simulink model "gm_sampleModel2005_4_sub_sub"  (R2023a)
settings: Solver=VariableStepAuto  StartTime=0.0  StopTime=10.0  RelTol=1e-3
libraries: hdlsllib x5, simulink x1
settings Model: Creator=user1  LastModifiedBy=user1
settings OptimizationCC: BlockReduction=off  ConditionallyExecuteInputs=off
settings DebuggingCC: InheritedTsInSrcMsg=none

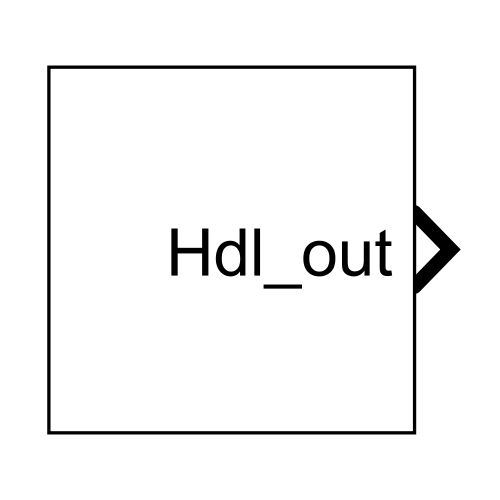
[thumbnail: Simulink's stored preview of the top-level diagram]
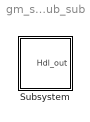
== system gm_sampleModel2005_4_sub_sub ==
  Subsystem : Subsystem

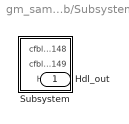
== system gm_sampleModel2005_4_sub_sub/Subsystem ==
  Subsystem : Subsystem
  Hdl_out : Outport  OutDataTypeStr=uint8

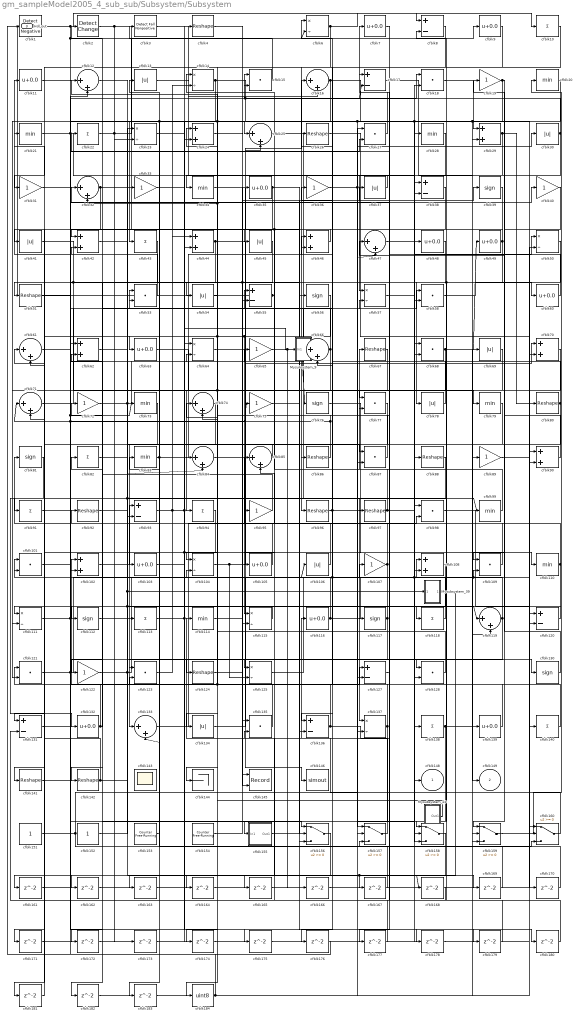
== system gm_sampleModel2005_4_sub_sub/Subsystem/Subsystem ==
  Mysubsystem_24 : Subsystem  TreatAsAtomicUnit=on  RTWFcnName=Mysubsystem_24
      settings: RTWFcnNameOpts=User specified  RTWFileNameOpts=Use function name
  Mysubsystem_39 : Subsystem  TreatAsAtomicUnit=on  RTWFcnName=Mysubsystem_39
      settings: RTWFcnNameOpts=User specified  RTWFileNameOpts=Use function name
  Mysubsystem_9 : Subsystem  TreatAsAtomicUnit=on  RTWFcnName=Mysubsystem_9
      settings: RTWFcnNameOpts=User specified  RTWFileNameOpts=Use function name
  cfblk1 : hdlsllib/Logic and Bit Operations/Detect Fall Negative  vinit=0  OutDataTypeStr=uint8
  cfblk{10,22,43,82,91,94,113,118,138,140} (10 alike) : Sum  Inputs=+  OutDataTypeStr=uint8
  cfblk{15,18,27,53,58,68,77,87,98,101,109,121,123,128,135} (15 alike) : DotProduct  OutDataTypeStr=uint8
  cfblk{24,29,42,44,46,62,70,90,102,108} (10 alike) : Sum  OutDataTypeStr=uint8
  cfblk{7,9,11,35,48..49,60,63,103,105,116,132,139} (13 alike) : Bias  Bias=0.0  SaturateOnIntegerOverflow=off
  cfblk{6,14,23,50,57,64,104,111,115,125,137} (11 alike) : Product  Inputs=*/  OutDataTypeStr=uint8  RndMeth=Zero  SaturateOnIntegerOverflow=on
  cfblk{13,30,37,41,45,54,69,78,106,134} (10 alike) : Abs  OutDataTypeStr=uint8  SaturateOnIntegerOverflow=off
  cfblk{19,31,33,36,40,65,72,75,89,95,107,122} (12 alike) : Gain  OutDataTypeStr=uint8
  cfblk{20..21,28,34,73,79,83,99,110,114} (10 alike) : MinMax  OutDataTypeStr=uint8
  cfblk{39,56,76,81,112,117,130} (7 alike) : Signum
  cfblk{12,16,25,32,47,61,66,71,74,84..85,119,133} (13 alike) : Sum  Inputs=|++  OutDataTypeStr=uint8
  cfblk{8,17,38,55,93,120,127,131,136} (9 alike) : Sum  Inputs=+-  OutDataTypeStr=uint8
  cfblk{4,26,51,67,80,86,88,92,96..97,124,141..142} (13 alike) : Reshape
  cfblk143 : Scope
      settings: Floating=on
  cfblk144 : Terminator
  cfblk145 : Record  FileSettingsInternal="{\"entries\":[{\"content\":{\"excelSettings\":{\"content\":{},\"type\":\"Streamout.ExcelSettings\"}},\"type\":\"Streamout.FileSettingStorage\",\"uuid\":\"\"}],\"packageUris\":[\"http:\\/\\/schema.mathworks.com\\/mf0\\/streamout_blocks\\/R2020a\"],\"version\":\"1.0\"}"  Layout=[1 1]  SignalsInternal="{\"entries\":[{\"content\":{\"signals\":[{\"content\":{\"blockPath\":[],\"dimensions\":[1],\"domain\":\"\",\"lineColor\":\"#a2142f\",\"plots\":[1],\"port\":1,\"signalID\":40483,\"signalName\":\"cfblk2\"},\"type\":\"RecordBlkView.Signal\",\"uuid\":\"\"},{\"content\":{\"blockPath\":[],\"dimensions\":[1],\"domain\":\"\",\"lineColor\":\"#139fff\",\"plots\":[1],\"port\":2,\"signalID\":40486,\"signalName\":\"cfblk45\"},\"type\":\"RecordBlkView.Signal\",\"uuid\":\"\"}]},\"type\":\"RecordBlkView.InputSignals\",\"uuid\":\"\"}],\"packageUris\":[\"http:\\/\\/schema.mathworks.com\\/mf0\\/streamout_blocks\\/R2020a\"],\"version\":\"1.0\"}"  VisualizationBindings="{\"xyplotplugin\":{\"info\":[{\"series\":[{\"bindingParametersList\":[{\"parameter\":\"X-Axis\",\"signalID\":40483,\"signalName\":\"cfblk2\"},{\"parameter\":\"Y-Axis\",\"signalID\":40486,\"signalName\":\"cfblk45\"}],\"seriesID\":27353}],\"subplotID\":1}]}}"  CompatibilityTag=XY  st=-1
  cfblk146 : ToWorkspace  VariableName=simout  SaveFormat=Timeseries  SampleTime=-1
  cfblk151 : Constant  OutDataTypeStr=uint8  SampleTime=-1
  cfblk152 : Constant  OutDataTypeStr=uint8  SampleTime=-1
  cfblk153 : hdlsllib/Sources/Counter Free-Running  NumBits=16  tsamp=-1
  cfblk154 : hdlsllib/Sources/Counter Free-Running  NumBits=16  tsamp=-1
  cfblk155 : Subsystem
      settings: LibrarySourceBlock=|
      | hdlsllib/Ports &
      | Subsystems/Subsystem
  cfblk{156..160} (5 alike) : Switch  OutDataTypeStr=uint8  SaturateOnIntegerOverflow=off  InputSameDT=off
  cfblk{161..183} (23 alike) : Delay  SampleTime=1
  cfblk184 : DataTypeConversion  OutDataTypeStr=uint8  SaturateOnIntegerOverflow=off  RndMeth=Floor
  cfblk2 : simulink/Logic and Bit Operations/Detect Change  vinit=0  OutDataTypeStr=uint8
      settings: LibrarySourceBlock=|
      | hdlsllib/Logic and Bit
      | Operations/Detect
      | Change
  cfblk3 : hdlsllib/Logic and Bit Operations/Detect Fall Nonpositive  vinit=0  OutDataTypeStr=uint8
  cfblk148 : Outport  OutDataTypeStr=uint8  VectorParamsAs1DForOutWhenUnconnected=off
  cfblk149 : Outport  Port=2  OutDataTypeStr=uint8  VectorParamsAs1DForOutWhenUnconnected=off
  Hdl_out : Outport  Port=3  OutDataTypeStr=uint8
  wires:
  cfblk137/1 -> cfblk172/1, cfblk102/1
  cfblk53/1 -> cfblk11/1
  cfblk123/1 -> cfblk44/1
  cfblk73/1 -> cfblk133/1
  cfblk97/1 -> cfblk110/1, cfblk67/1
  cfblk136/1 -> cfblk42/2, cfblk32/1
  cfblk6/1 -> cfblk10/1, cfblk31/1
  cfblk74/1 -> cfblk142/1
  cfblk8/1 -> cfblk96/1
  cfblk22/1 -> cfblk23/2, cfblk9/1
  cfblk49/1 -> cfblk42/1, cfblk78/1
  cfblk14/1 -> cfblk43/1, cfblk17/2, cfblk47/2, cfblk149/1
  cfblk25/1 -> cfblk137/1
  cfblk112/1 -> cfblk84/2, Mysubsystem_39/1(In1)
  cfblk115/1 -> cfblk111/1
  cfblk81/1 -> cfblk132/1
  cfblk29/1 -> cfblk66/2, cfblk80/1
  cfblk87/1 -> cfblk32/2, cfblk12/1
  cfblk11/1 -> cfblk25/1
  cfblk21/1 -> cfblk179/1, cfblk148/1
  cfblk64/1 -> cfblk16/1
  cfblk131/1 -> cfblk58/1
  cfblk125/1 -> cfblk108/1
  cfblk44/1 -> cfblk51/1, cfblk146/1
  cfblk84/1 -> cfblk46/1
  cfblk102/1 -> cfblk93/1
  cfblk66/1 -> cfblk2/1, cfblk94/1
  cfblk37/1 -> cfblk34/1
  cfblk78/1 -> cfblk26/1
  cfblk83/1 -> cfblk183/1, cfblk25/2
  cfblk26/1 -> cfblk140/1
  cfblk134/1 -> cfblk107/1
  cfblk132/1 -> cfblk62/2, cfblk101/1
  cfblk41/1 -> cfblk66/1, cfblk79/1
  cfblk106/1 -> cfblk81/1
  cfblk121/1 -> cfblk48/1, cfblk75/1, cfblk27/2
  cfblk3/1 -> cfblk57/1
  cfblk128/1 -> cfblk74/1
  cfblk33/1 -> cfblk117/1, cfblk108/2
  cfblk85/1 -> cfblk84/1
  cfblk13/1 -> cfblk16/2
  cfblk159/1 -> cfblk20/1
  cfblk152/1 -> cfblk103/1
  cfblk104/1 -> cfblk125/2, cfblk70/1
  cfblk68/1 -> cfblk121/2, cfblk49/1
  cfblk135/1 -> cfblk82/1
  cfblk118/1 -> cfblk21/1
  cfblk160/1 -> cfblk116/1
  cfblk105/1 -> cfblk83/1
  cfblk16/1 -> cfblk160/2, cfblk44/2, cfblk144/1
  cfblk47/1 -> cfblk88/1
  cfblk42/1 -> cfblk156/1
  cfblk99/1 -> cfblk14/1
  cfblk65/1 -> cfblk166/1, cfblk76/1
  cfblk67/1 -> cfblk134/1, cfblk91/1
  cfblk138/1 -> cfblk165/1, cfblk69/1
  cfblk56/1 -> cfblk115/1, cfblk174/1, cfblk61/2
  cfblk133/1 -> cfblk85/1
  cfblk43/1 -> cfblk122/1
  cfblk103/1 -> cfblk64/1
  cfblk57/1 -> cfblk50/1
  cfblk19/1 -> cfblk109/1, cfblk68/2, cfblk133/2, cfblk111/2
  cfblk109/1 -> cfblk85/2
  cfblk76/1 -> cfblk138/1
  cfblk31/1 -> cfblk45/1
  cfblk24/1 -> cfblk135/1
  cfblk140/1 -> cfblk61/1, cfblk24/1
  cfblk17/1 -> cfblk89/1
  cfblk155/1(Out1) -> cfblk37/1
  cfblk27/1 -> cfblk7/1
  cfblk9/1 -> cfblk54/1
  cfblk111/1 -> cfblk127/2, cfblk18/1, cfblk4/1
  cfblk96/1 -> cfblk36/1, cfblk139/1
  cfblk70/1 -> cfblk93/2
  cfblk80/1 -> cfblk171/1, cfblk53/2
  cfblk69/1 -> cfblk158/1
  cfblk157/1 -> cfblk114/1
  cfblk93/1 -> cfblk14/2, cfblk65/1, cfblk168/1, cfblk167/1
  cfblk98/1 -> cfblk120/2
  cfblk50/1 -> cfblk128/1, cfblk155/1(In1)
  cfblk122/1 -> cfblk169/1, cfblk28/1
  cfblk127/1 -> cfblk17/1
  cfblk79/1 -> cfblk95/1
  cfblk117/1 -> cfblk156/3, cfblk92/1
  cfblk114/1 -> cfblk98/2
  cfblk94/1 -> cfblk141/1
  cfblk4/1 -> cfblk38/2
  cfblk116/1 -> cfblk71/2, cfblk18/2, cfblk90/2
  cfblk77/1 -> cfblk136/1
  cfblk71/1 -> cfblk55/1
  cfblk40/1 -> cfblk159/1
  cfblk130/1 -> cfblk47/1
  cfblk82/1 -> cfblk87/1
  cfblk54/1 -> cfblk124/1
  cfblk2/1 -> cfblk173/1, cfblk145/1
  cfblk30/1 -> cfblk15/2, cfblk137/2
  cfblk12/1 -> cfblk119/1, cfblk113/1
  cfblk58/1 -> cfblk60/1
  cfblk35/1 -> cfblk180/1, cfblk63/1
  cfblk10/1 -> cfblk86/1
  cfblk95/1 -> cfblk72/1
  cfblk72/1 -> cfblk118/1, cfblk57/2
  cfblk28/1 -> cfblk158/2
  cfblk51/1 -> cfblk40/1
  cfblk151/1 -> cfblk160/3, cfblk27/1
  cfblk63/1 -> cfblk157/1
  cfblk86/1 -> cfblk71/1, cfblk15/1
  cfblk60/1 -> cfblk22/1
  cfblk154/1 -> cfblk39/1
  cfblk34/1 -> cfblk56/1
  cfblk124/1 -> cfblk35/1
  cfblk62/1 -> cfblk115/2, cfblk99/1
  cfblk120/1 -> cfblk112/1
  cfblk18/1 -> cfblk29/1
  cfblk107/1 -> cfblk104/2, cfblk6/1
  cfblk90/1 -> cfblk19/1
  cfblk55/1 -> Hdl_out/1, cfblk105/1
  cfblk113/1 -> cfblk130/1, Mysubsystem_9/1(In1)
  cfblk91/1 -> cfblk156/2
  cfblk36/1 -> cfblk158/3, cfblk30/1
  cfblk61/1 -> cfblk102/2
  cfblk141/1 -> cfblk127/1
  cfblk119/1 -> cfblk123/1, cfblk109/2, cfblk74/2
  cfblk110/1 -> cfblk128/2, cfblk53/1
  cfblk139/1 -> cfblk46/2, cfblk106/1
  cfblk153/1 -> cfblk13/1
  cfblk46/1 -> cfblk41/1
  cfblk142/1 -> cfblk121/1, cfblk23/1
  cfblk1/1 -> cfblk8/1, cfblk55/2, cfblk6/2
  cfblk15/1 -> cfblk3/1
  cfblk92/1 -> cfblk97/1
  cfblk45/1 -> cfblk182/1, cfblk145/2
  cfblk38/1 -> cfblk104/1, cfblk125/1
  cfblk101/1 -> cfblk73/1, cfblk64/2
  cfblk20/1 -> cfblk29/2, cfblk77/1
  cfblk32/1 -> cfblk33/1, cfblk131/1
  cfblk39/1 -> cfblk136/2
  cfblk88/1 -> cfblk161/1
  cfblk161/1 -> cfblk12/2
  cfblk162/1 -> cfblk98/1
  cfblk108/1 -> cfblk163/1
  cfblk163/1 -> cfblk68/1
  cfblk158/1 -> cfblk164/1
  cfblk164/1 -> cfblk120/1
  cfblk165/1 -> cfblk70/2
  cfblk166/1 -> cfblk119/2
  cfblk167/1 -> cfblk123/2
  cfblk168/1 -> cfblk131/2
  cfblk169/1 -> cfblk157/3
  cfblk89/1 -> cfblk170/1
  cfblk170/1 -> cfblk38/1
  cfblk171/1 -> cfblk24/2
  cfblk172/1 -> cfblk58/2
  cfblk173/1 -> cfblk157/2
  cfblk174/1 -> cfblk159/2
  cfblk23/1 -> cfblk175/1
  cfblk175/1 -> cfblk90/1
  cfblk48/1 -> cfblk176/1
  cfblk176/1 -> cfblk1/1
  cfblk7/1 -> cfblk177/1
  cfblk177/1 -> cfblk135/2
  cfblk75/1 -> cfblk178/1
  cfblk178/1 -> cfblk50/2
  cfblk179/1 -> cfblk8/2
  cfblk180/1 -> cfblk77/2
  cfblk156/1 -> cfblk181/1
  cfblk181/1 -> cfblk101/2
  cfblk182/1 -> cfblk160/1
  cfblk183/1 -> cfblk159/3
  cfblk184/1 -> cfblk87/2, cfblk62/1
  Mysubsystem_24/1(Out1) -> cfblk184/1
  Mysubsystem_39/1(Out1) -> cfblk162/1

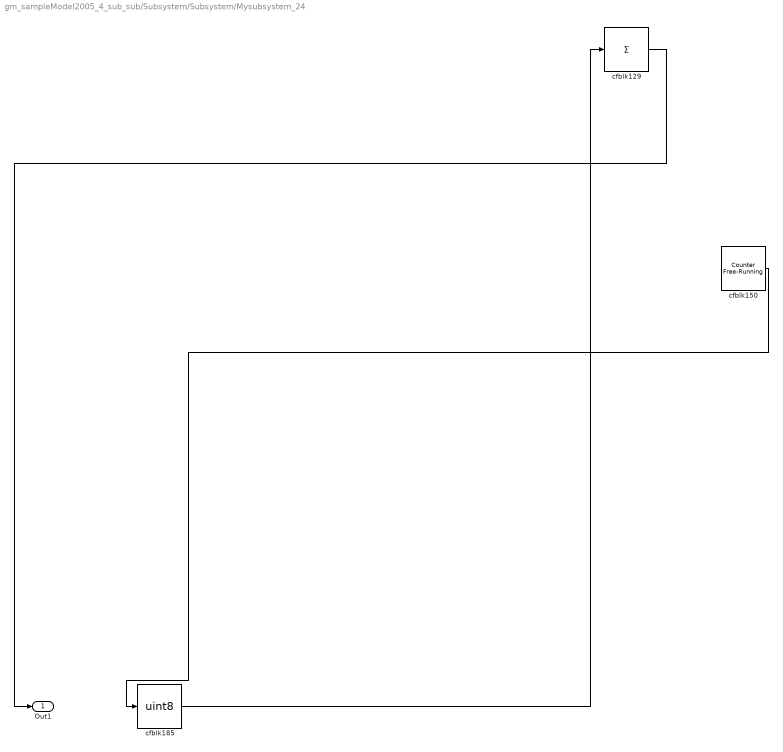
== system gm_sampleModel2005_4_sub_sub/Subsystem/Subsystem/Mysubsystem_24 ==
  cfblk129 : Sum  Inputs=+
  cfblk150 : hdlsllib/Sources/Counter Free-Running  NumBits=16  tsamp=-1
  cfblk185 : DataTypeConversion  OutDataTypeStr=uint8  SaturateOnIntegerOverflow=off  RndMeth=Floor
  Out1 : Outport
  wires:
  cfblk129/1 -> Out1/1
  cfblk150/1 -> cfblk185/1
  cfblk185/1 -> cfblk129/1

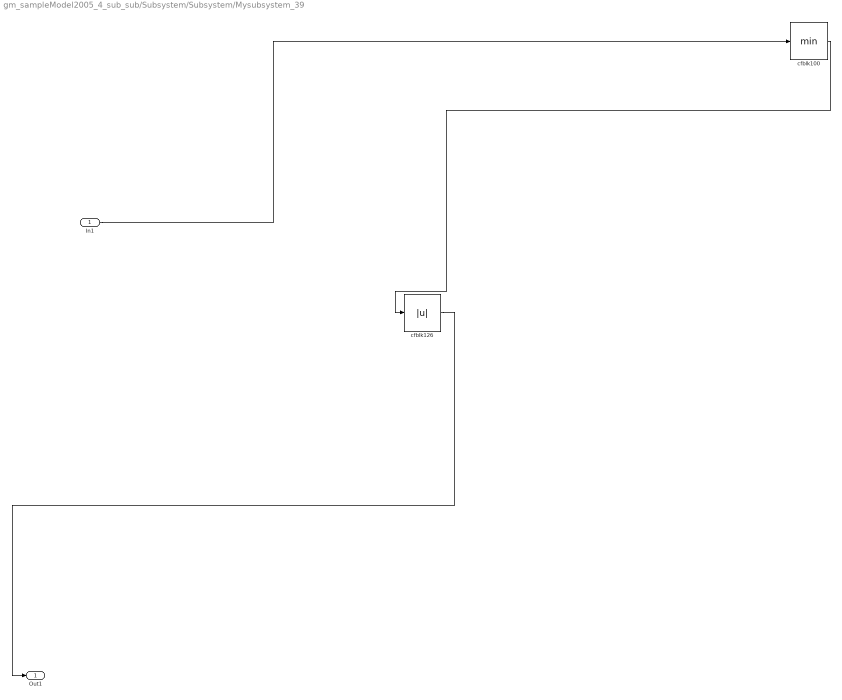
== system gm_sampleModel2005_4_sub_sub/Subsystem/Subsystem/Mysubsystem_39 ==
  In1 : Inport
  cfblk100 : MinMax
  cfblk126 : Abs  SaturateOnIntegerOverflow=off
  Out1 : Outport
  wires:
  cfblk126/1 -> Out1/1
  In1/1 -> cfblk100/1
  cfblk100/1 -> cfblk126/1

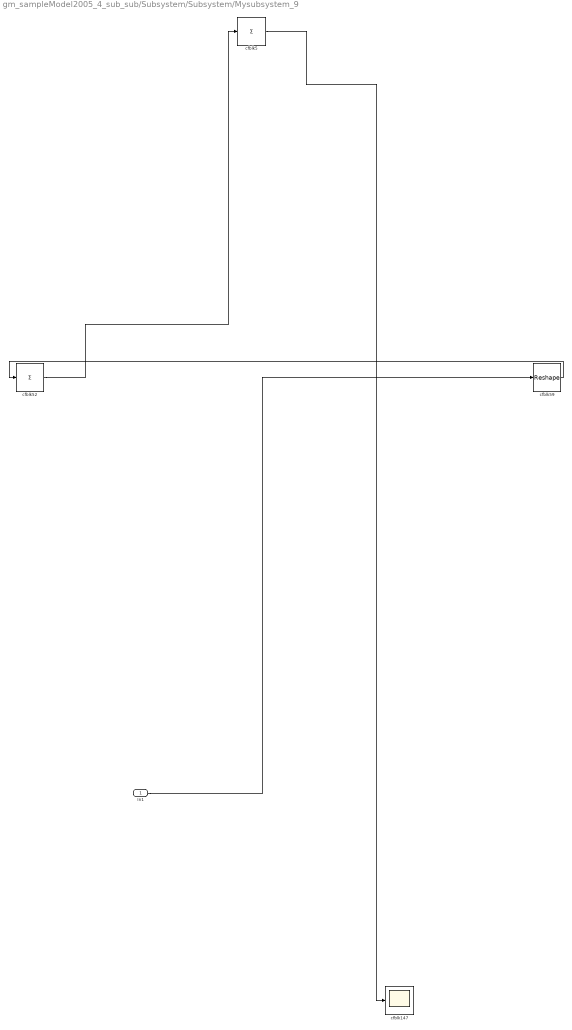
== system gm_sampleModel2005_4_sub_sub/Subsystem/Subsystem/Mysubsystem_9 ==
  In1 : Inport
  cfblk147 : Scope
  cfblk5 : Sum  Inputs=+
  cfblk52 : Sum  Inputs=+
  cfblk59 : Reshape
  wires:
  cfblk5/1 -> cfblk147/1
  cfblk59/1 -> cfblk52/1
  cfblk52/1 -> cfblk5/1
  In1/1 -> cfblk59/1

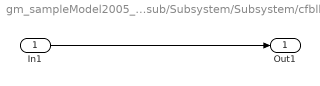
== system gm_sampleModel2005_4_sub_sub/Subsystem/Subsystem/cfblk155 ==
  In1 : Inport
  Out1 : Outport
  wires:
  In1/1 -> Out1/1
